simulink library "controls_module_lib"  (R2024b)
settings: Solver=VariableStepAuto  StartTime=0.0  StopTime=10.0  RelTol=1e-3
undefined symbols (not defined in the file): j, S_NOM, SNOM, VLL, VLL_NOM
libraries: simulink x14
(part 1 of 2)
settings Model: Creator=HussamAlatrash  LastModifiedBy=HussamAlatrash

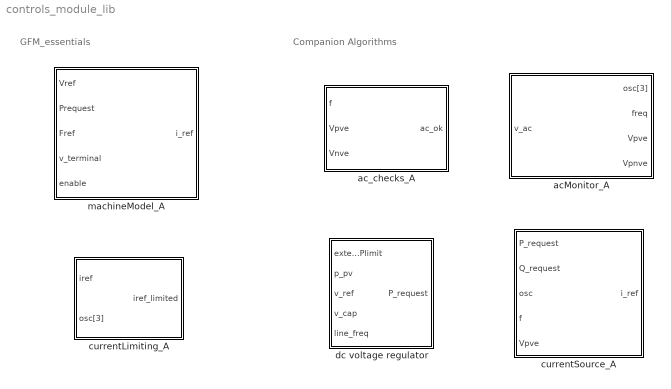
== system controls_module_lib ==
  note: Companion Algorithms
  note: GFM_essentials
  acMonitor_A : Subsystem  mask{VllRated=VLL, nominalFrequency=60}
      mask prompts: VllRated "Rated line-to-line voltage (V)"; nominalFrequency "Nominal line frequency (Hz)"
  ac_checks_A : Subsystem  mask{VllRated=1, nominalFrequency=60, tRequalify=5, T_CNTL=1e-3}
      mask prompts: VllRated "Rated line-to-line voltage (V)"; nominalFrequency "Nominal line frequency (Hz)"; tRequalify "Reconnection time (sec)"; T_CNTL "Operating sample time"
  currentLimiting_A : Subsystem  mask{IRated=SNOM/(sqrt(3)*VLL), RmsLimit=1.5, peakSoftLimit=2.6, peakHardLimit=3.5}
      mask prompts: IRated "Rated current (A)"; RmsLimit "Rms Current Limit (pu)"; peakSoftLimit "Soft peak limit (pu)"; peakHardLimit "Hard peak limit (pu)"
  currentSource_A : Subsystem  mask{VllRated=VLL_NOM, SRated=S_NOM, nominalFrequency=60, Plimit=1, Qlimit=0.5}
      mask prompts: VllRated "Rated line-to-line voltage (V)"; SRated "Rated power (VA)"; nominalFrequency "Nominal line frequency (Hz)"; Plimit "Real power request limit (pu)"; Qlimit "Reactive power request limit (pu)"
  dc voltage regulator : Subsystem  mask{kpFast=300, kpSlow=0.0, pRequestMax=1.2*S_NOM, pRequestMin=-1.2*S_NOM, pLimitExternalMinimum=0.05*SNOM}
      mask prompts: kpFast "Proportional gain - fast path (W/V)"; kpSlow "Proportional gain - filtered (slow) path (W/V)"; pRequestMax "Maximum power request (W)"; pRequestMin "Minimum power request (W)"; pLimitExternalMinimum "Minimum value for external power limit (W)"
  machineModel_A : Subsystem  mask{SRated=SNOM, VllRated=VLL, nominalFrequency=60, inertialConstant=2, kDroop=1, kDamper=2, Xs=0.2, rs=0.03}
      mask prompts: SRated "Rated power (VA)"; VllRated "Rated Voltage (Volts, line-to-line)"; nominalFrequency "Nominal frequency (Hz)"; inertialConstant "Inertial constant (seconds)"; kDroop "Droop gain (pu/Hz)"; kDamper "Damper gain (pu/Hz)"; Xs "Stator reactance (pu)"; rs "Stator resistance (pu)"

== system controls_module_lib/acMonitor_A ==
  v_ac : Inport
  Analyzer_V : Subsystem
  PLL_3ph : Subsystem
  to_pu : Gain  Gain=1/VllRated
  osc[3] : Outport
  freq : Outport  Port=2
  Vpve : Outport  Port=3
  Vpnve : Outport  Port=4
  wires:
  PLL_3ph/1(osc[3]) -> Analyzer_V/2(osc[3]), osc[3]/1
  PLL_3ph/2(freq) -> freq/1
  v_ac/1 -> Analyzer_V/1(in[3]), to_pu/1
  to_pu/1 -> PLL_3ph/1(ref)
  Analyzer_V/3(Pve) -> Vpve/1
  Analyzer_V/4(Nve) -> Vpnve/1

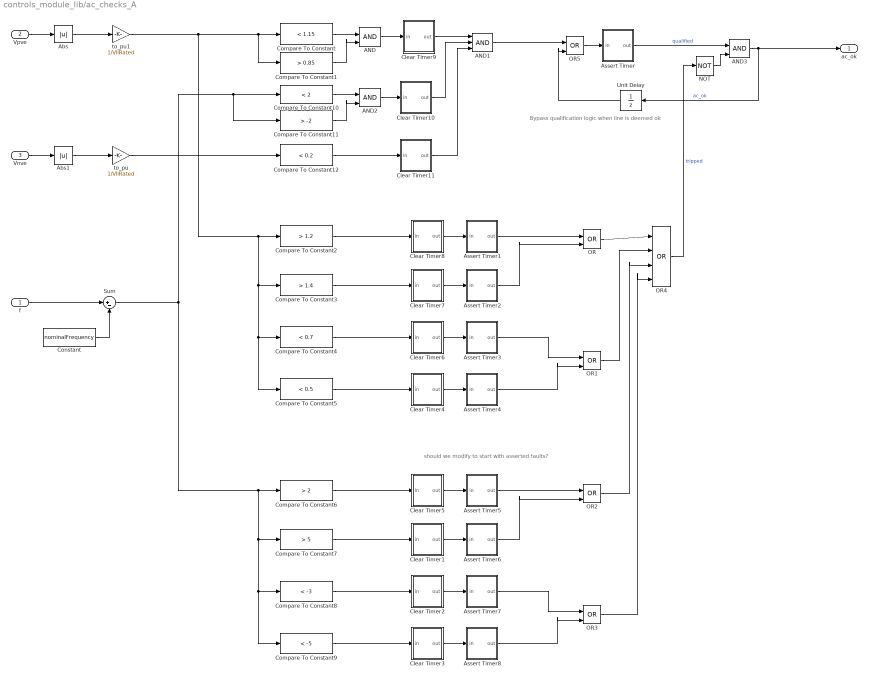
== system controls_module_lib/ac_checks_A ==
  note: should we modify to start with asserted faults?
  note: Bypass qualification logic when line is deemed ok
  f : Inport
  Vpve : Inport  Port=2
  Vnve : Inport  Port=3
  AND : Logic  IconShape=distinctive  AllPortsSameDT=off  OutDataTypeStr=boolean
  AND1 : Logic  Inputs=3  IconShape=distinctive  AllPortsSameDT=off  OutDataTypeStr=boolean
  AND2 : Logic  IconShape=distinctive  AllPortsSameDT=off  OutDataTypeStr=boolean
  AND3 : Logic  IconShape=distinctive  AllPortsSameDT=off  OutDataTypeStr=boolean
  Abs : Abs  SaturateOnIntegerOverflow=off
  Abs1 : Abs  SaturateOnIntegerOverflow=off
  Assert Timer : Subsystem  mask{T_STEP=T_CNTL, TIMEOUT=tRequalify}
      mask prompts: T_STEP "Time step"
  Assert Timer1 : Subsystem  mask{T_STEP=T_CNTL, TIMEOUT=60}
      mask prompts: T_STEP "Time step"
  Assert Timer2 : Subsystem  mask{T_STEP=T_CNTL, TIMEOUT=10}
      mask prompts: T_STEP "Time step"
  Assert Timer3 : Subsystem  mask{T_STEP=T_CNTL, TIMEOUT=60}
      mask prompts: T_STEP "Time step"
  Assert Timer4 : Subsystem  mask{T_STEP=T_CNTL, TIMEOUT=10}
      mask prompts: T_STEP "Time step"
  Assert Timer5 : Subsystem  mask{T_STEP=T_CNTL, TIMEOUT=60}
      mask prompts: T_STEP "Time step"
  Assert Timer6 : Subsystem  mask{T_STEP=T_CNTL, TIMEOUT=10}
      mask prompts: T_STEP "Time step"
  Assert Timer7 : Subsystem  mask{T_STEP=T_CNTL, TIMEOUT=60}
      mask prompts: T_STEP "Time step"
  Assert Timer8 : Subsystem  mask{T_STEP=T_CNTL, TIMEOUT=10}
      mask prompts: T_STEP "Time step"
  Clear Timer1 : Subsystem  mask{T_STEP=T_CNTL, TIMEOUT=0.1, TIMER_INIT=0.1}
      mask prompts: T_STEP "Time step"; TIMER_INIT "Timer initial value"
  Clear Timer10 : Subsystem  mask{T_STEP=T_CNTL, TIMEOUT=0.1, TIMER_INIT=0}
      mask prompts: T_STEP "Time step"; TIMER_INIT "Timer initial value"
  Clear Timer11 : Subsystem  mask{T_STEP=T_CNTL, TIMEOUT=0.1, TIMER_INIT=0}
      mask prompts: T_STEP "Time step"; TIMER_INIT "Timer initial value"
  Clear Timer2 : Subsystem  mask{T_STEP=T_CNTL, TIMEOUT=0.1, TIMER_INIT=0.1}
      mask prompts: T_STEP "Time step"; TIMER_INIT "Timer initial value"
  Clear Timer3 : Subsystem  mask{T_STEP=T_CNTL, TIMEOUT=0.1, TIMER_INIT=0.1}
      mask prompts: T_STEP "Time step"; TIMER_INIT "Timer initial value"
  Clear Timer4 : Subsystem  mask{T_STEP=T_CNTL, TIMEOUT=0.1, TIMER_INIT=0}
      mask prompts: T_STEP "Time step"; TIMER_INIT "Timer initial value"
  Clear Timer5 : Subsystem  mask{T_STEP=T_CNTL, TIMEOUT=0.1, TIMER_INIT=0.1}
      mask prompts: T_STEP "Time step"; TIMER_INIT "Timer initial value"
  Clear Timer6 : Subsystem  mask{T_STEP=T_CNTL, TIMEOUT=0.1, TIMER_INIT=0}
      mask prompts: T_STEP "Time step"; TIMER_INIT "Timer initial value"
  Clear Timer7 : Subsystem  mask{T_STEP=T_CNTL, TIMEOUT=0.1, TIMER_INIT=0}
      mask prompts: T_STEP "Time step"; TIMER_INIT "Timer initial value"
  Clear Timer8 : Subsystem  mask{T_STEP=T_CNTL, TIMEOUT=0.1, TIMER_INIT=0}
      mask prompts: T_STEP "Time step"; TIMER_INIT "Timer initial value"
  Clear Timer9 : Subsystem  mask{T_STEP=T_CNTL, TIMEOUT=0.1, TIMER_INIT=0}
      mask prompts: T_STEP "Time step"; TIMER_INIT "Timer initial value"
  Compare To Constant : simulink/Logic and Bit Operations/Compare To Constant  relop=<  const=1.15  OutDataTypeStr=boolean
  Compare To Constant1 : simulink/Logic and Bit Operations/Compare To Constant  relop=>  const=0.85  OutDataTypeStr=boolean
  Compare To Constant10 : simulink/Logic and Bit Operations/Compare To Constant  relop=<  const=2  OutDataTypeStr=boolean
  Compare To Constant11 : simulink/Logic and Bit Operations/Compare To Constant  relop=>  const=-2  OutDataTypeStr=boolean
  Compare To Constant12 : simulink/Logic and Bit Operations/Compare To Constant  relop=<  const=0.2  OutDataTypeStr=boolean
  Compare To Constant2 : simulink/Logic and Bit Operations/Compare To Constant  relop=>  const=1.2  OutDataTypeStr=boolean
  Compare To Constant3 : simulink/Logic and Bit Operations/Compare To Constant  relop=>  const=1.4  OutDataTypeStr=boolean
  Compare To Constant4 : simulink/Logic and Bit Operations/Compare To Constant  relop=<  const=0.7  OutDataTypeStr=boolean
  Compare To Constant5 : simulink/Logic and Bit Operations/Compare To Constant  relop=<  const=0.5  OutDataTypeStr=boolean
  Compare To Constant6 : simulink/Logic and Bit Operations/Compare To Constant  relop=>  const=2  OutDataTypeStr=boolean
  Compare To Constant7 : simulink/Logic and Bit Operations/Compare To Constant  relop=>  const=5  OutDataTypeStr=boolean
  Compare To Constant8 : simulink/Logic and Bit Operations/Compare To Constant  relop=<  const=-3  OutDataTypeStr=boolean
  Compare To Constant9 : simulink/Logic and Bit Operations/Compare To Constant  relop=<  const=-5  OutDataTypeStr=boolean
  Constant : Constant  Value=nominalFrequency
  NOT : Logic  Operator=NOT  IconShape=distinctive  AllPortsSameDT=off  OutDataTypeStr=boolean
  OR{,1..3,5} (5 alike) : Logic  Operator=OR  IconShape=distinctive  AllPortsSameDT=off  OutDataTypeStr=boolean
  OR4 : Logic  Operator=OR  Inputs=4  IconShape=distinctive  AllPortsSameDT=off  OutDataTypeStr=boolean
  Sum : Sum  Inputs=|+-
  Unit Delay : UnitDelay  SampleTime=T_CNTL  HasFrameUpgradeWarning=on
  to_pu : Gain  Gain=1/VllRated
  to_pu1 : Gain  Gain=1/VllRated
  ac_ok : Outport
  wires:
  OR2/1 -> OR4/3
  AND3/1 -> ac_ok/1, Unit Delay/1  "ac_ok"
  Clear Timer4/1(out) -> Assert Timer4/1(in)
  OR/1 -> OR4/1
  Clear Timer9/1(out) -> AND1/1
  Compare To Constant10/1 -> AND2/1
  Assert Timer2/1(out) -> OR/2
  OR4/1 -> NOT/1  "tripped"
  Sum/1 -> Compare To Constant6/1, Compare To Constant7/1, Compare To Constant8/1, Compare To Constant9/1, Compare To Constant10/1, Compare To Constant11/1
  Clear Timer7/1(out) -> Assert Timer2/1(in)
  Vpve/1 -> Abs/1
  Clear Timer3/1(out) -> Assert Timer8/1(in)
  Clear Timer10/1(out) -> AND1/2
  Compare To Constant7/1 -> Clear Timer1/1(in)
  Compare To Constant5/1 -> Clear Timer4/1(in)
  AND/1 -> Clear Timer9/1(in)
  Clear Timer2/1(out) -> Assert Timer7/1(in)
  OR1/1 -> OR4/2
  Compare To Constant8/1 -> Clear Timer2/1(in)
  AND1/1 -> OR5/1
  Clear Timer6/1(out) -> Assert Timer3/1(in)
  Assert Timer6/1(out) -> OR2/2
  Compare To Constant4/1 -> Clear Timer6/1(in)
  Compare To Constant11/1 -> AND2/2
  Compare To Constant9/1 -> Clear Timer3/1(in)
  AND2/1 -> Clear Timer10/1(in)
  Compare To Constant3/1 -> Clear Timer7/1(in)
  Compare To Constant/1 -> AND/1
  Assert Timer3/1(out) -> OR1/1
  NOT/1 -> AND3/2
  Vnve/1 -> Abs1/1
  Assert Timer8/1(out) -> OR3/2
  Assert Timer7/1(out) -> OR3/1
  Clear Timer8/1(out) -> Assert Timer1/1(in)
  Clear Timer1/1(out) -> Assert Timer6/1(in)
  Compare To Constant6/1 -> Clear Timer5/1(in)
  Clear Timer5/1(out) -> Assert Timer5/1(in)
  Assert Timer5/1(out) -> OR2/1
  Assert Timer4/1(out) -> OR1/2
  OR3/1 -> OR4/4
  Assert Timer/1(out) -> AND3/1  "qualified"
  Compare To Constant1/1 -> AND/2
  Compare To Constant2/1 -> Clear Timer8/1(in)
  OR5/1 -> Assert Timer/1(in)
  Clear Timer11/1(out) -> AND1/3
  Compare To Constant12/1 -> Clear Timer11/1(in)
  Assert Timer1/1(out) -> OR/1
  Unit Delay/1 -> OR5/2
  Abs/1 -> to_pu1/1
  Abs1/1 -> to_pu/1
  to_pu1/1 -> Compare To Constant1/1, Compare To Constant/1, Compare To Constant5/1, Compare To Constant4/1, Compare To Constant3/1, Compare To Constant2/1
  to_pu/1 -> Compare To Constant12/1
  f/1 -> Sum/1
  Constant/1 -> Sum/2

== system controls_module_lib/currentLimiting_A ==
  iref : Inport
  osc[3] : Inport  Port=2
  Analyzer_I : Subsystem
  Sum2 : Sum  Inputs=|+-
  excess_sink : Subsystem
  soft_saturation : Subsystem  mask{soft_limit=peakSoftLimit*IRated, hard_limit=peakHardLimit*IRated}
      mask prompts: soft_limit "Soft limit"; hard_limit "Hard limit"
  iref_limited : Outport
  wires:
  Sum2/1 -> soft_saturation/1(in)
  osc[3]/1 -> excess_sink/2(osc[3]), Analyzer_I/2(osc[3])
  iref/1 -> Sum2/1, Analyzer_I/1(in[3])
  excess_sink/1(i_excess[3]) -> Sum2/2
  Analyzer_I/1(fund[3]) -> excess_sink/1(I_total[3])  "I_total[3]"
  soft_saturation/1(out) -> iref_limited/1

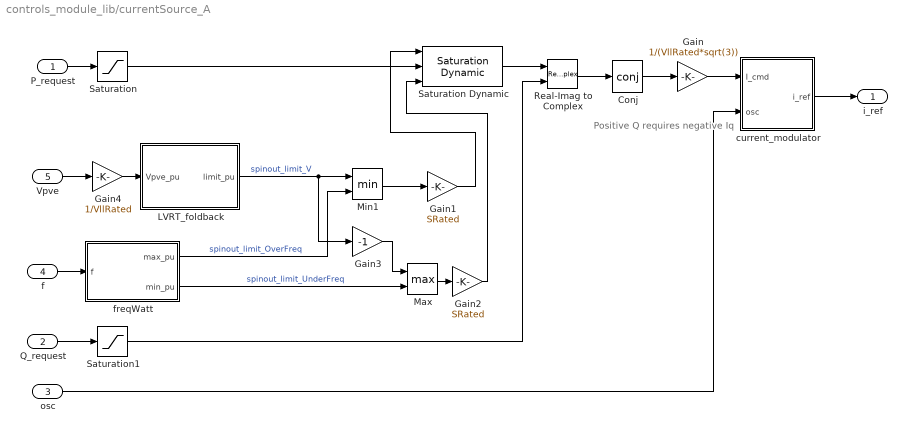
== system controls_module_lib/currentSource_A ==
  note: Positive Q requires negative Iq
  P_request : Inport
  Q_request : Inport  Port=2
  osc : Inport  Port=3
  f : Inport  Port=4
  Vpve : Inport  Port=5
  Conj : Math  Operator=conj
  Gain : Gain  Gain=1/(VllRated*sqrt(3))
  Gain1 : Gain  Gain=SRated
  Gain2 : Gain  Gain=SRated
  Gain3 : Gain  Gain=-1
  Gain4 : Gain  Gain=1/VllRated
  LVRT_foldback : Subsystem
  Max : MinMax  Function=max  Inputs=2
  Min1 : MinMax  Inputs=2
  Real-Imag to Complex : RealImagToComplex
  Saturation : Saturate  UpperLimit=Plimit*SRated  LowerLimit=-Plimit*SRated
  Saturation Dynamic : simulink/Discontinuities/Saturation Dynamic  OutMin=[]  OutMax=[]  OutDataTypeStr=Inherit: Same as second input  OutDataType=fixdt(1, 16)  OutScaling=2^-10  DoSatur=off
  Saturation1 : Saturate  UpperLimit=Qlimit*SRated  LowerLimit=-Qlimit*SRated
  current_modulator : Subsystem
  freqWatt : Subsystem
  i_ref : Outport
  wires:
  LVRT_foldback/1(limit_pu) -> Min1/1, Gain3/1  "spinout_limit_V"
  Vpve/1 -> Gain4/1
  Min1/1 -> Gain1/1
  f/1 -> freqWatt/1(f)
  freqWatt/1(max_pu) -> Min1/2  "spinout_limit_OverFreq"
  current_modulator/1(i_ref) -> i_ref/1
  Q_request/1 -> Saturation1/1
  P_request/1 -> Saturation/1
  osc/1 -> current_modulator/2(osc)
  Gain4/1 -> LVRT_foldback/1(Vpve_pu)
  Saturation Dynamic/1 -> Real-Imag to Complex/1
  Gain1/1 -> Saturation Dynamic/1
  Real-Imag to Complex/1 -> Conj/1
  Conj/1 -> Gain/1
  Gain/1 -> current_modulator/1(I_cmd)
  Saturation/1 -> Saturation Dynamic/2
  Saturation1/1 -> Real-Imag to Complex/2
  Max/1 -> Gain2/1
  freqWatt/2(min_pu) -> Max/2  "spinout_limit_UnderFreq"
  Gain2/1 -> Saturation Dynamic/3
  Gain3/1 -> Max/1

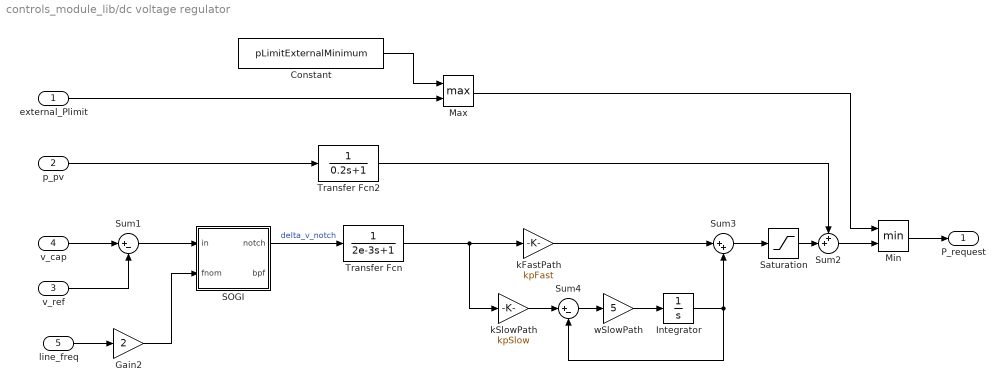
== system controls_module_lib/dc voltage regulator ==
  external_Plimit : Inport
  p_pv : Inport  Port=2
  v_ref : Inport  Port=3
  v_cap : Inport  Port=4
  line_freq : Inport  Port=5
  Constant : Constant  Value=pLimitExternalMinimum
  Gain2 : Gain  Gain=2
  Integrator : Integrator  LimitOutput=on  UpperSaturationLimit=0.4  LowerSaturationLimit=-0.1
  Max : MinMax  Function=max  Inputs=2
  Min : MinMax  Inputs=2
  SOGI : Subsystem
  Saturation : Saturate  UpperLimit=pRequestMax  LowerLimit=pRequestMin
  Sum1 : Sum  Inputs=|+-
  Sum2 : Sum  Inputs=++|
  Sum3 : Sum  Inputs=|++
  Sum4 : Sum  Inputs=|+-
  Transfer Fcn : TransferFcn  Denominator=[2e-3 1]
  Transfer Fcn2 : TransferFcn  Denominator=[0.2 1]
  kFastPath : Gain  Gain=kpFast
  kSlowPath : Gain  Gain=kpSlow
  wSlowPath : Gain  Gain=5
  P_request : Outport
  wires:
  Constant/1 -> Max/1
  external_Plimit/1 -> Max/2
  Max/1 -> Min/1
  Min/1 -> P_request/1
  v_ref/1 -> Sum1/2
  Sum2/1 -> Min/2
  Gain2/1 -> SOGI/2(fnom)
  SOGI/1(notch) -> Transfer Fcn/1  "delta_v_notch"
  v_cap/1 -> Sum1/1
  p_pv/1 -> Transfer Fcn2/1
  Transfer Fcn/1 -> kSlowPath/1, kFastPath/1
  kFastPath/1 -> Sum3/1
  Sum3/1 -> Saturation/1
  kSlowPath/1 -> Sum4/1
  Transfer Fcn2/1 -> Sum2/1
  line_freq/1 -> Gain2/1
  Integrator/1 -> Sum4/2, Sum3/2
  Saturation/1 -> Sum2/2
  wSlowPath/1 -> Integrator/1
  Sum4/1 -> wSlowPath/1
  Sum1/1 -> SOGI/1(in)

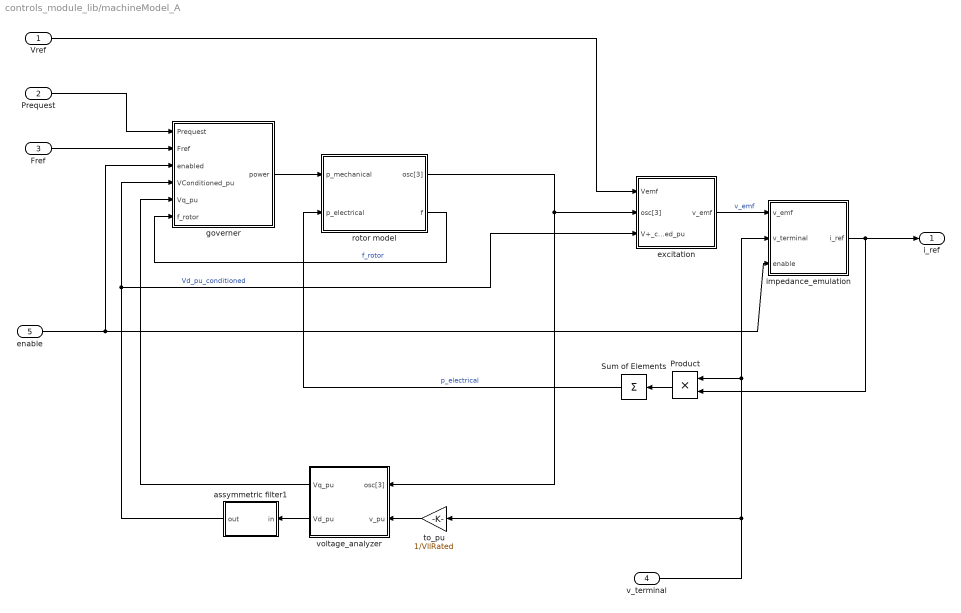
== system controls_module_lib/machineModel_A ==
  Vref : Inport
  Prequest : Inport  Port=2
  Fref : Inport  Port=3
  v_terminal : Inport  Port=4
  enable : Inport  Port=5
  Product : Product
  Sum of Elements : Sum  Inputs=+
  assymmetric filter1 : Subsystem
  excitation : Subsystem
  governer : Subsystem
  impedance_emulation : Subsystem
  rotor model : Subsystem
  to_pu : Gain  Gain=1/VllRated
  voltage_analyzer : Subsystem
  i_ref : Outport
  wires:
  excitation/1(v_emf) -> impedance_emulation/1(v_emf)  "v_emf"
  rotor model/1(osc[3]) -> excitation/2(osc[3]), voltage_analyzer/1(osc[3])
  Product/1 -> Sum of Elements/1
  Sum of Elements/1 -> rotor model/2(p_electrical)  "p_electrical"
  governer/1(power) -> rotor model/1(p_mechanical)
  voltage_analyzer/2(Vd_pu) -> assymmetric filter1/1(in)
  Prequest/1 -> governer/1(Prequest)
  impedance_emulation/1(i_ref) -> i_ref/1, Product/2
  to_pu/1 -> voltage_analyzer/2(v_pu)
  v_terminal/1 -> to_pu/1, impedance_emulation/2(v_terminal), Product/1
  voltage_analyzer/1(Vq_pu) -> governer/5(Vq_pu)
  rotor model/2(f) -> governer/6(f_rotor)  "f_rotor"
  assymmetric filter1/1(out) -> excitation/3(V+_conditioned_pu), governer/4(VConditioned_pu)  "Vd_pu_conditioned"
  enable/1 -> governer/3(enabled), impedance_emulation/3(enable)
  Fref/1 -> governer/2(Fref)
  Vref/1 -> excitation/1(Vemf)

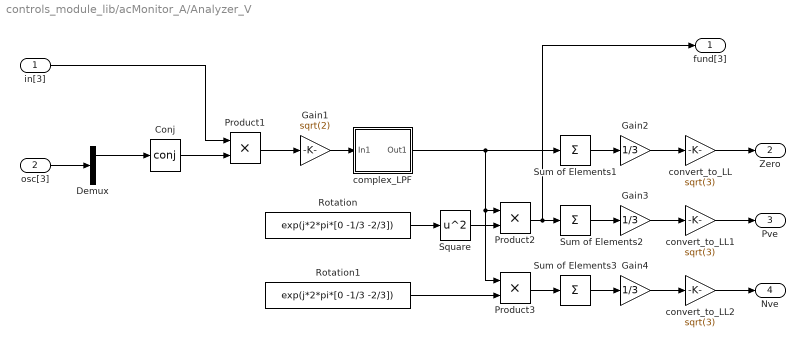
== system controls_module_lib/acMonitor_A/Analyzer_V ==
  in[3] : Inport
  osc[3] : Inport  Port=2
  Conj : Math  Operator=conj
  Demux : Demux  Outputs=3
  Gain1 : Gain  Gain=sqrt(2)
  Gain2 : Gain  Gain=1/3
  Gain3 : Gain  Gain=1/3
  Gain4 : Gain  Gain=1/3
  Product1 : Product
  Product2 : Product
  Product3 : Product
  Rotation : Constant  Value=exp(j*2*pi*[0 -1/3 -2/3])
  Rotation1 : Constant  Value=exp(j*2*pi*[0 -1/3 -2/3])
  Square : Math  Operator=square
  Sum of Elements1 : Sum  Inputs=+
  Sum of Elements2 : Sum  Inputs=+
  Sum of Elements3 : Sum  Inputs=+
  complex_LPF : Subsystem  mask{tau=0.05}
      mask prompts: tau "Time constant"
  convert_to_LL : Gain  Gain=sqrt(3)
  convert_to_LL1 : Gain  Gain=sqrt(3)
  convert_to_LL2 : Gain  Gain=sqrt(3)
  fund[3] : Outport
  Zero : Outport  Port=2
  Pve : Outport  Port=3
  Nve : Outport  Port=4
  wires:
  Gain4/1 -> convert_to_LL2/1
  Product2/1 -> fund[3]/1, Sum of Elements2/1
  complex_LPF/1(Out1) -> Product3/1, Product2/1, Sum of Elements1/1
  Product1/1 -> Gain1/1
  Product3/1 -> Sum of Elements3/1
  Gain1/1 -> complex_LPF/1(In1)
  Demux/1 -> Conj/1
  Rotation/1 -> Square/1
  Rotation1/1 -> Product3/2
  Sum of Elements2/1 -> Gain3/1
  Conj/1 -> Product1/2
  Sum of Elements1/1 -> Gain2/1
  Square/1 -> Product2/2
  Sum of Elements3/1 -> Gain4/1
  osc[3]/1 -> Demux/1
  Gain3/1 -> convert_to_LL1/1
  Gain2/1 -> convert_to_LL/1
  in[3]/1 -> Product1/1
  convert_to_LL/1 -> Zero/1
  convert_to_LL1/1 -> Pve/1
  convert_to_LL2/1 -> Nve/1

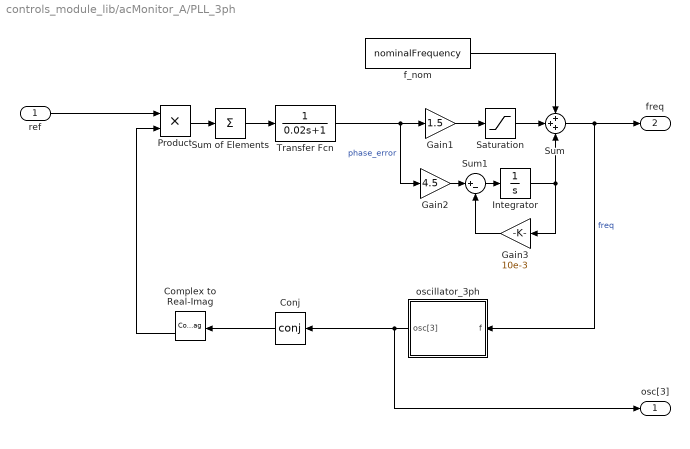
== system controls_module_lib/acMonitor_A/PLL_3ph ==
  ref : Inport
  Complex to Real-Imag : ComplexToRealImag
  Conj : Math  Operator=conj
  Gain1 : Gain  Gain=1.5
  Gain2 : Gain  Gain=4.5
  Gain3 : Gain  Gain=10e-3
  Integrator : Integrator  LimitOutput=on  UpperSaturationLimit=5  LowerSaturationLimit=-5
  Product : Product
  Saturation : Saturate  UpperLimit=5  LowerLimit=-5
  Sum : Sum  Inputs=+++
  Sum of Elements : Sum  Inputs=+
  Sum1 : Sum  Inputs=|+-
  Transfer Fcn : TransferFcn  Denominator=[0.02 1]
  f_nom : Constant  Value=nominalFrequency
  oscillator_3ph : Subsystem
  osc[3] : Outport
  freq : Outport  Port=2
  wires:
  f_nom/1 -> Sum/1
  Gain3/1 -> Sum1/2
  Sum of Elements/1 -> Transfer Fcn/1
  Transfer Fcn/1 -> Gain2/1, Gain1/1  "phase_error"
  Saturation/1 -> Sum/2
  Product/1 -> Sum of Elements/1
  Sum/1 -> freq/1, oscillator_3ph/1(f)  "freq"
  oscillator_3ph/1(osc[3]) -> Conj/1, osc[3]/1
  Gain2/1 -> Sum1/1
  Complex to Real-Imag/2 -> Product/2
  Sum1/1 -> Integrator/1
  Integrator/1 -> Gain3/1, Sum/3
  ref/1 -> Product/1
  Conj/1 -> Complex to Real-Imag/1
  Gain1/1 -> Saturation/1

== system controls_module_lib/ac_checks_A/Assert Timer ==
  in : Inport
  Constant : Constant  Value=T_STEP
  Constant1 : Constant  Value=0
  Constant2 : Constant  Value=TIMEOUT
  Min2 : MinMax  Inputs=2
  Relational Operator : RelationalOperator  Operator=>  OutDataTypeStr=boolean  RndMeth=Simplest  InputSameDT=off
  Sum2 : Sum  Inputs=|++
  Switch : Switch  Criteria=u2 > Threshold  SaturateOnIntegerOverflow=off  InputSameDT=off
  Unit Delay : UnitDelay  SampleTime=T_STEP  HasFrameUpgradeWarning=on
  out : Outport
  wires:
  Sum2/1 -> Relational Operator/1, Min2/1
  Constant2/1 -> Min2/2, Relational Operator/2
  Constant/1 -> Sum2/1
  Min2/1 -> Switch/1
  Constant1/1 -> Switch/3
  Unit Delay/1 -> Sum2/2
  in/1 -> Switch/2
  Switch/1 -> Unit Delay/1
  Relational Operator/1 -> out/1

== system controls_module_lib/ac_checks_A/Assert Timer1 ==
  in : Inport
  Constant : Constant  Value=T_STEP
  Constant1 : Constant  Value=0
  Constant2 : Constant  Value=TIMEOUT
  Min2 : MinMax  Inputs=2
  Relational Operator : RelationalOperator  Operator=>  OutDataTypeStr=boolean  RndMeth=Simplest  InputSameDT=off
  Sum2 : Sum  Inputs=|++
  Switch : Switch  Criteria=u2 > Threshold  SaturateOnIntegerOverflow=off  InputSameDT=off
  Unit Delay : UnitDelay  SampleTime=T_STEP  HasFrameUpgradeWarning=on
  out : Outport
  wires:
  Relational Operator/1 -> out/1
  Switch/1 -> Unit Delay/1
  in/1 -> Switch/2
  Unit Delay/1 -> Sum2/2
  Constant1/1 -> Switch/3
  Min2/1 -> Switch/1
  Constant/1 -> Sum2/1
  Constant2/1 -> Relational Operator/2, Min2/2
  Sum2/1 -> Min2/1, Relational Operator/1

== system controls_module_lib/ac_checks_A/Assert Timer2 ==
  in : Inport
  Constant : Constant  Value=T_STEP
  Constant1 : Constant  Value=0
  Constant2 : Constant  Value=TIMEOUT
  Min2 : MinMax  Inputs=2
  Relational Operator : RelationalOperator  Operator=>  OutDataTypeStr=boolean  RndMeth=Simplest  InputSameDT=off
  Sum2 : Sum  Inputs=|++
  Switch : Switch  Criteria=u2 > Threshold  SaturateOnIntegerOverflow=off  InputSameDT=off
  Unit Delay : UnitDelay  SampleTime=T_STEP  HasFrameUpgradeWarning=on
  out : Outport
  wires:
  Sum2/1 -> Relational Operator/1, Min2/1
  Constant2/1 -> Min2/2, Relational Operator/2
  Constant/1 -> Sum2/1
  Min2/1 -> Switch/1
  Constant1/1 -> Switch/3
  Unit Delay/1 -> Sum2/2
  in/1 -> Switch/2
  Switch/1 -> Unit Delay/1
  Relational Operator/1 -> out/1

== system controls_module_lib/ac_checks_A/Assert Timer3 ==
  in : Inport
  Constant : Constant  Value=T_STEP
  Constant1 : Constant  Value=0
  Constant2 : Constant  Value=TIMEOUT
  Min2 : MinMax  Inputs=2
  Relational Operator : RelationalOperator  Operator=>  OutDataTypeStr=boolean  RndMeth=Simplest  InputSameDT=off
  Sum2 : Sum  Inputs=|++
  Switch : Switch  Criteria=u2 > Threshold  SaturateOnIntegerOverflow=off  InputSameDT=off
  Unit Delay : UnitDelay  SampleTime=T_STEP  HasFrameUpgradeWarning=on
  out : Outport
  wires:
  Relational Operator/1 -> out/1
  Switch/1 -> Unit Delay/1
  in/1 -> Switch/2
  Unit Delay/1 -> Sum2/2
  Constant1/1 -> Switch/3
  Min2/1 -> Switch/1
  Constant/1 -> Sum2/1
  Constant2/1 -> Relational Operator/2, Min2/2
  Sum2/1 -> Min2/1, Relational Operator/1

== system controls_module_lib/ac_checks_A/Assert Timer4 ==
  in : Inport
  Constant : Constant  Value=T_STEP
  Constant1 : Constant  Value=0
  Constant2 : Constant  Value=TIMEOUT
  Min2 : MinMax  Inputs=2
  Relational Operator : RelationalOperator  Operator=>  OutDataTypeStr=boolean  RndMeth=Simplest  InputSameDT=off
  Sum2 : Sum  Inputs=|++
  Switch : Switch  Criteria=u2 > Threshold  SaturateOnIntegerOverflow=off  InputSameDT=off
  Unit Delay : UnitDelay  SampleTime=T_STEP  HasFrameUpgradeWarning=on
  out : Outport
  wires:
  Sum2/1 -> Relational Operator/1, Min2/1
  Constant2/1 -> Min2/2, Relational Operator/2
  Constant/1 -> Sum2/1
  Min2/1 -> Switch/1
  Constant1/1 -> Switch/3
  Unit Delay/1 -> Sum2/2
  in/1 -> Switch/2
  Switch/1 -> Unit Delay/1
  Relational Operator/1 -> out/1

== system controls_module_lib/ac_checks_A/Assert Timer5 ==
  in : Inport
  Constant : Constant  Value=T_STEP
  Constant1 : Constant  Value=0
  Constant2 : Constant  Value=TIMEOUT
  Min2 : MinMax  Inputs=2
  Relational Operator : RelationalOperator  Operator=>  OutDataTypeStr=boolean  RndMeth=Simplest  InputSameDT=off
  Sum2 : Sum  Inputs=|++
  Switch : Switch  Criteria=u2 > Threshold  SaturateOnIntegerOverflow=off  InputSameDT=off
  Unit Delay : UnitDelay  SampleTime=T_STEP  HasFrameUpgradeWarning=on
  out : Outport
  wires:
  Sum2/1 -> Relational Operator/1, Min2/1
  Constant2/1 -> Min2/2, Relational Operator/2
  Constant/1 -> Sum2/1
  Min2/1 -> Switch/1
  Constant1/1 -> Switch/3
  Unit Delay/1 -> Sum2/2
  in/1 -> Switch/2
  Switch/1 -> Unit Delay/1
  Relational Operator/1 -> out/1

== system controls_module_lib/ac_checks_A/Assert Timer6 ==
  in : Inport
  Constant : Constant  Value=T_STEP
  Constant1 : Constant  Value=0
  Constant2 : Constant  Value=TIMEOUT
  Min2 : MinMax  Inputs=2
  Relational Operator : RelationalOperator  Operator=>  OutDataTypeStr=boolean  RndMeth=Simplest  InputSameDT=off
  Sum2 : Sum  Inputs=|++
  Switch : Switch  Criteria=u2 > Threshold  SaturateOnIntegerOverflow=off  InputSameDT=off
  Unit Delay : UnitDelay  SampleTime=T_STEP  HasFrameUpgradeWarning=on
  out : Outport
  wires:
  Relational Operator/1 -> out/1
  Switch/1 -> Unit Delay/1
  in/1 -> Switch/2
  Unit Delay/1 -> Sum2/2
  Constant1/1 -> Switch/3
  Min2/1 -> Switch/1
  Constant/1 -> Sum2/1
  Constant2/1 -> Relational Operator/2, Min2/2
  Sum2/1 -> Min2/1, Relational Operator/1

== system controls_module_lib/ac_checks_A/Assert Timer7 ==
  in : Inport
  Constant : Constant  Value=T_STEP
  Constant1 : Constant  Value=0
  Constant2 : Constant  Value=TIMEOUT
  Min2 : MinMax  Inputs=2
  Relational Operator : RelationalOperator  Operator=>  OutDataTypeStr=boolean  RndMeth=Simplest  InputSameDT=off
  Sum2 : Sum  Inputs=|++
  Switch : Switch  Criteria=u2 > Threshold  SaturateOnIntegerOverflow=off  InputSameDT=off
  Unit Delay : UnitDelay  SampleTime=T_STEP  HasFrameUpgradeWarning=on
  out : Outport
  wires:
  Sum2/1 -> Relational Operator/1, Min2/1
  Constant2/1 -> Min2/2, Relational Operator/2
  Constant/1 -> Sum2/1
  Min2/1 -> Switch/1
  Constant1/1 -> Switch/3
  Unit Delay/1 -> Sum2/2
  in/1 -> Switch/2
  Switch/1 -> Unit Delay/1
  Relational Operator/1 -> out/1

== system controls_module_lib/ac_checks_A/Assert Timer8 ==
  in : Inport
  Constant : Constant  Value=T_STEP
  Constant1 : Constant  Value=0
  Constant2 : Constant  Value=TIMEOUT
  Min2 : MinMax  Inputs=2
  Relational Operator : RelationalOperator  Operator=>  OutDataTypeStr=boolean  RndMeth=Simplest  InputSameDT=off
  Sum2 : Sum  Inputs=|++
  Switch : Switch  Criteria=u2 > Threshold  SaturateOnIntegerOverflow=off  InputSameDT=off
  Unit Delay : UnitDelay  SampleTime=T_STEP  HasFrameUpgradeWarning=on
  out : Outport
  wires:
  Relational Operator/1 -> out/1
  Switch/1 -> Unit Delay/1
  in/1 -> Switch/2
  Unit Delay/1 -> Sum2/2
  Constant1/1 -> Switch/3
  Min2/1 -> Switch/1
  Constant/1 -> Sum2/1
  Constant2/1 -> Relational Operator/2, Min2/2
  Sum2/1 -> Min2/1, Relational Operator/1

== system controls_module_lib/ac_checks_A/Clear Timer1 ==
  in : Inport
  Constant : Constant  Value=T_STEP
  Constant1 : Constant  Value=0
  Constant2 : Constant  Value=TIMEOUT
  Min2 : MinMax  Function=max  Inputs=2
  Relational Operator : RelationalOperator  Operator=>  OutDataTypeStr=boolean  RndMeth=Simplest  InputSameDT=off
  Sum2 : Sum  Inputs=|-+
  Switch : Switch  Criteria=u2 > Threshold  SaturateOnIntegerOverflow=off  InputSameDT=off
  Unit Delay : UnitDelay  InitialCondition=TIMER_INIT  SampleTime=T_STEP  HasFrameUpgradeWarning=on
  out : Outport
  wires:
  Constant2/1 -> Switch/1
  Sum2/1 -> Relational Operator/1, Min2/1
  Constant/1 -> Sum2/1
  Min2/1 -> Switch/3
  Constant1/1 -> Min2/2, Relational Operator/2
  Unit Delay/1 -> Sum2/2
  in/1 -> Switch/2
  Switch/1 -> Unit Delay/1
  Relational Operator/1 -> out/1

== system controls_module_lib/ac_checks_A/Clear Timer10 ==
  in : Inport
  Constant : Constant  Value=T_STEP
  Constant1 : Constant  Value=0
  Constant2 : Constant  Value=TIMEOUT
  Min2 : MinMax  Function=max  Inputs=2
  Relational Operator : RelationalOperator  Operator=>  OutDataTypeStr=boolean  RndMeth=Simplest  InputSameDT=off
  Sum2 : Sum  Inputs=|-+
  Switch : Switch  Criteria=u2 > Threshold  SaturateOnIntegerOverflow=off  InputSameDT=off
  Unit Delay : UnitDelay  InitialCondition=TIMER_INIT  SampleTime=T_STEP  HasFrameUpgradeWarning=on
  out : Outport
  wires:
  Constant2/1 -> Switch/1
  Sum2/1 -> Relational Operator/1, Min2/1
  Constant/1 -> Sum2/1
  Min2/1 -> Switch/3
  Constant1/1 -> Min2/2, Relational Operator/2
  Unit Delay/1 -> Sum2/2
  in/1 -> Switch/2
  Switch/1 -> Unit Delay/1
  Relational Operator/1 -> out/1

== system controls_module_lib/ac_checks_A/Clear Timer11 ==
  in : Inport
  Constant : Constant  Value=T_STEP
  Constant1 : Constant  Value=0
  Constant2 : Constant  Value=TIMEOUT
  Min2 : MinMax  Function=max  Inputs=2
  Relational Operator : RelationalOperator  Operator=>  OutDataTypeStr=boolean  RndMeth=Simplest  InputSameDT=off
  Sum2 : Sum  Inputs=|-+
  Switch : Switch  Criteria=u2 > Threshold  SaturateOnIntegerOverflow=off  InputSameDT=off
  Unit Delay : UnitDelay  InitialCondition=TIMER_INIT  SampleTime=T_STEP  HasFrameUpgradeWarning=on
  out : Outport
  wires:
  Relational Operator/1 -> out/1
  Switch/1 -> Unit Delay/1
  in/1 -> Switch/2
  Unit Delay/1 -> Sum2/2
  Constant1/1 -> Relational Operator/2, Min2/2
  Min2/1 -> Switch/3
  Constant/1 -> Sum2/1
  Sum2/1 -> Min2/1, Relational Operator/1
  Constant2/1 -> Switch/1

== system controls_module_lib/ac_checks_A/Clear Timer2 ==
  in : Inport
  Constant : Constant  Value=T_STEP
  Constant1 : Constant  Value=0
  Constant2 : Constant  Value=TIMEOUT
  Min2 : MinMax  Function=max  Inputs=2
  Relational Operator : RelationalOperator  Operator=>  OutDataTypeStr=boolean  RndMeth=Simplest  InputSameDT=off
  Sum2 : Sum  Inputs=|-+
  Switch : Switch  Criteria=u2 > Threshold  SaturateOnIntegerOverflow=off  InputSameDT=off
  Unit Delay : UnitDelay  InitialCondition=TIMER_INIT  SampleTime=T_STEP  HasFrameUpgradeWarning=on
  out : Outport
  wires:
  Relational Operator/1 -> out/1
  Switch/1 -> Unit Delay/1
  in/1 -> Switch/2
  Unit Delay/1 -> Sum2/2
  Constant1/1 -> Relational Operator/2, Min2/2
  Min2/1 -> Switch/3
  Constant/1 -> Sum2/1
  Sum2/1 -> Min2/1, Relational Operator/1
  Constant2/1 -> Switch/1

== system controls_module_lib/ac_checks_A/Clear Timer3 ==
  in : Inport
  Constant : Constant  Value=T_STEP
  Constant1 : Constant  Value=0
  Constant2 : Constant  Value=TIMEOUT
  Min2 : MinMax  Function=max  Inputs=2
  Relational Operator : RelationalOperator  Operator=>  OutDataTypeStr=boolean  RndMeth=Simplest  InputSameDT=off
  Sum2 : Sum  Inputs=|-+
  Switch : Switch  Criteria=u2 > Threshold  SaturateOnIntegerOverflow=off  InputSameDT=off
  Unit Delay : UnitDelay  InitialCondition=TIMER_INIT  SampleTime=T_STEP  HasFrameUpgradeWarning=on
  out : Outport
  wires:
  Constant2/1 -> Switch/1
  Sum2/1 -> Relational Operator/1, Min2/1
  Constant/1 -> Sum2/1
  Min2/1 -> Switch/3
  Constant1/1 -> Min2/2, Relational Operator/2
  Unit Delay/1 -> Sum2/2
  in/1 -> Switch/2
  Switch/1 -> Unit Delay/1
  Relational Operator/1 -> out/1

== system controls_module_lib/ac_checks_A/Clear Timer4 ==
  in : Inport
  Constant : Constant  Value=T_STEP
  Constant1 : Constant  Value=0
  Constant2 : Constant  Value=TIMEOUT
  Min2 : MinMax  Function=max  Inputs=2
  Relational Operator : RelationalOperator  Operator=>  OutDataTypeStr=boolean  RndMeth=Simplest  InputSameDT=off
  Sum2 : Sum  Inputs=|-+
  Switch : Switch  Criteria=u2 > Threshold  SaturateOnIntegerOverflow=off  InputSameDT=off
  Unit Delay : UnitDelay  InitialCondition=TIMER_INIT  SampleTime=T_STEP  HasFrameUpgradeWarning=on
  out : Outport
  wires:
  Relational Operator/1 -> out/1
  Switch/1 -> Unit Delay/1
  in/1 -> Switch/2
  Unit Delay/1 -> Sum2/2
  Constant1/1 -> Relational Operator/2, Min2/2
  Min2/1 -> Switch/3
  Constant/1 -> Sum2/1
  Sum2/1 -> Min2/1, Relational Operator/1
  Constant2/1 -> Switch/1

== system controls_module_lib/ac_checks_A/Clear Timer5 ==
  in : Inport
  Constant : Constant  Value=T_STEP
  Constant1 : Constant  Value=0
  Constant2 : Constant  Value=TIMEOUT
  Min2 : MinMax  Function=max  Inputs=2
  Relational Operator : RelationalOperator  Operator=>  OutDataTypeStr=boolean  RndMeth=Simplest  InputSameDT=off
  Sum2 : Sum  Inputs=|-+
  Switch : Switch  Criteria=u2 > Threshold  SaturateOnIntegerOverflow=off  InputSameDT=off
  Unit Delay : UnitDelay  InitialCondition=TIMER_INIT  SampleTime=T_STEP  HasFrameUpgradeWarning=on
  out : Outport
  wires:
  Relational Operator/1 -> out/1
  Switch/1 -> Unit Delay/1
  in/1 -> Switch/2
  Unit Delay/1 -> Sum2/2
  Constant1/1 -> Relational Operator/2, Min2/2
  Min2/1 -> Switch/3
  Constant/1 -> Sum2/1
  Sum2/1 -> Min2/1, Relational Operator/1
  Constant2/1 -> Switch/1

== system controls_module_lib/ac_checks_A/Clear Timer6 ==
  in : Inport
  Constant : Constant  Value=T_STEP
  Constant1 : Constant  Value=0
  Constant2 : Constant  Value=TIMEOUT
  Min2 : MinMax  Function=max  Inputs=2
  Relational Operator : RelationalOperator  Operator=>  OutDataTypeStr=boolean  RndMeth=Simplest  InputSameDT=off
  Sum2 : Sum  Inputs=|-+
  Switch : Switch  Criteria=u2 > Threshold  SaturateOnIntegerOverflow=off  InputSameDT=off
  Unit Delay : UnitDelay  InitialCondition=TIMER_INIT  SampleTime=T_STEP  HasFrameUpgradeWarning=on
  out : Outport
  wires:
  Constant2/1 -> Switch/1
  Sum2/1 -> Relational Operator/1, Min2/1
  Constant/1 -> Sum2/1
  Min2/1 -> Switch/3
  Constant1/1 -> Min2/2, Relational Operator/2
  Unit Delay/1 -> Sum2/2
  in/1 -> Switch/2
  Switch/1 -> Unit Delay/1
  Relational Operator/1 -> out/1

== system controls_module_lib/ac_checks_A/Clear Timer7 ==
  in : Inport
  Constant : Constant  Value=T_STEP
  Constant1 : Constant  Value=0
  Constant2 : Constant  Value=TIMEOUT
  Min2 : MinMax  Function=max  Inputs=2
  Relational Operator : RelationalOperator  Operator=>  OutDataTypeStr=boolean  RndMeth=Simplest  InputSameDT=off
  Sum2 : Sum  Inputs=|-+
  Switch : Switch  Criteria=u2 > Threshold  SaturateOnIntegerOverflow=off  InputSameDT=off
  Unit Delay : UnitDelay  InitialCondition=TIMER_INIT  SampleTime=T_STEP  HasFrameUpgradeWarning=on
  out : Outport
  wires:
  Relational Operator/1 -> out/1
  Switch/1 -> Unit Delay/1
  in/1 -> Switch/2
  Unit Delay/1 -> Sum2/2
  Constant1/1 -> Relational Operator/2, Min2/2
  Min2/1 -> Switch/3
  Constant/1 -> Sum2/1
  Sum2/1 -> Min2/1, Relational Operator/1
  Constant2/1 -> Switch/1

== system controls_module_lib/ac_checks_A/Clear Timer8 ==
  in : Inport
  Constant : Constant  Value=T_STEP
  Constant1 : Constant  Value=0
  Constant2 : Constant  Value=TIMEOUT
  Min2 : MinMax  Function=max  Inputs=2
  Relational Operator : RelationalOperator  Operator=>  OutDataTypeStr=boolean  RndMeth=Simplest  InputSameDT=off
  Sum2 : Sum  Inputs=|-+
  Switch : Switch  Criteria=u2 > Threshold  SaturateOnIntegerOverflow=off  InputSameDT=off
  Unit Delay : UnitDelay  InitialCondition=TIMER_INIT  SampleTime=T_STEP  HasFrameUpgradeWarning=on
  out : Outport
  wires:
  Constant2/1 -> Switch/1
  Sum2/1 -> Relational Operator/1, Min2/1
  Constant/1 -> Sum2/1
  Min2/1 -> Switch/3
  Constant1/1 -> Min2/2, Relational Operator/2
  Unit Delay/1 -> Sum2/2
  in/1 -> Switch/2
  Switch/1 -> Unit Delay/1
  Relational Operator/1 -> out/1

== system controls_module_lib/ac_checks_A/Clear Timer9 ==
  in : Inport
  Constant : Constant  Value=T_STEP
  Constant1 : Constant  Value=0
  Constant2 : Constant  Value=TIMEOUT
  Min2 : MinMax  Function=max  Inputs=2
  Relational Operator : RelationalOperator  Operator=>  OutDataTypeStr=boolean  RndMeth=Simplest  InputSameDT=off
  Sum2 : Sum  Inputs=|-+
  Switch : Switch  Criteria=u2 > Threshold  SaturateOnIntegerOverflow=off  InputSameDT=off
  Unit Delay : UnitDelay  InitialCondition=TIMER_INIT  SampleTime=T_STEP  HasFrameUpgradeWarning=on
  out : Outport
  wires:
  Relational Operator/1 -> out/1
  Switch/1 -> Unit Delay/1
  in/1 -> Switch/2
  Unit Delay/1 -> Sum2/2
  Constant1/1 -> Relational Operator/2, Min2/2
  Min2/1 -> Switch/3
  Constant/1 -> Sum2/1
  Sum2/1 -> Min2/1, Relational Operator/1
  Constant2/1 -> Switch/1

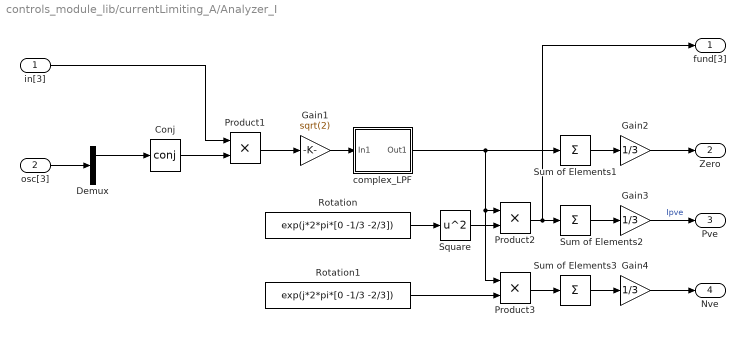
== system controls_module_lib/currentLimiting_A/Analyzer_I ==
  in[3] : Inport
  osc[3] : Inport  Port=2
  Conj : Math  Operator=conj
  Demux : Demux  Outputs=3
  Gain1 : Gain  Gain=sqrt(2)
  Gain2 : Gain  Gain=1/3
  Gain3 : Gain  Gain=1/3
  Gain4 : Gain  Gain=1/3
  Product1 : Product
  Product2 : Product
  Product3 : Product
  Rotation : Constant  Value=exp(j*2*pi*[0 -1/3 -2/3])
  Rotation1 : Constant  Value=exp(j*2*pi*[0 -1/3 -2/3])
  Square : Math  Operator=square
  Sum of Elements1 : Sum  Inputs=+
  Sum of Elements2 : Sum  Inputs=+
  Sum of Elements3 : Sum  Inputs=+
  complex_LPF : Subsystem  mask{tau=0.02}
      mask prompts: tau "Time constant"
  fund[3] : Outport
  Zero : Outport  Port=2
  Pve : Outport  Port=3
  Nve : Outport  Port=4
  wires:
  in[3]/1 -> Product1/1
  Gain2/1 -> Zero/1
  Gain3/1 -> Pve/1  "Ipve"
  osc[3]/1 -> Demux/1
  Sum of Elements3/1 -> Gain4/1
  Square/1 -> Product2/2
  Sum of Elements1/1 -> Gain2/1
  Conj/1 -> Product1/2
  Sum of Elements2/1 -> Gain3/1
  Rotation1/1 -> Product3/2
  Rotation/1 -> Square/1
  Demux/1 -> Conj/1
  Gain1/1 -> complex_LPF/1(In1)
  Product3/1 -> Sum of Elements3/1
  Product1/1 -> Gain1/1
  complex_LPF/1(Out1) -> Sum of Elements1/1, Product2/1, Product3/1
  Product2/1 -> Sum of Elements2/1, fund[3]/1
  Gain4/1 -> Nve/1

== system controls_module_lib/currentLimiting_A/excess_sink ==
  I_total[3] : Inport
  osc[3] : Inport  Port=2
  Complex to Real-Imag : ComplexToRealImag
  Ilimit : Constant  Value=RmsLimit * IRated
  Product3 : Product
  RMS Limiter : Subsystem
  Sum : Sum  Inputs=|-+
  sqrt(2) : Gain  Gain=sqrt(2)
  i_excess[3] : Outport
  wires:
  sqrt(2)/1 -> Product3/2
  Product3/1 -> Complex to Real-Imag/1
  I_total[3]/1 -> RMS Limiter/2(I[3]), Sum/2
  Sum/1 -> Product3/1  "Iexcess[3]"
  Complex to Real-Imag/1 -> i_excess[3]/1
  osc[3]/1 -> sqrt(2)/1
  Ilimit/1 -> RMS Limiter/1(limit)
  RMS Limiter/1(I_limited[3]) -> Sum/1

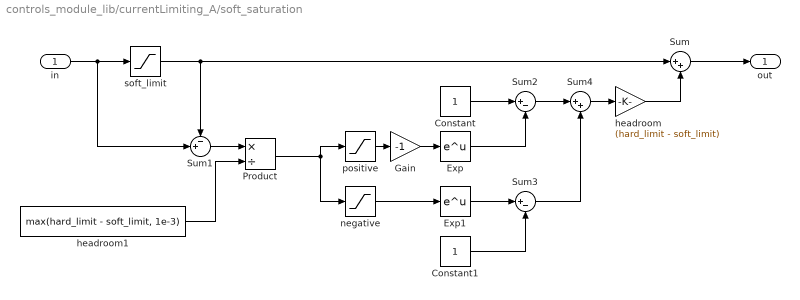
== system controls_module_lib/currentLimiting_A/soft_saturation ==
  in : Inport
  Constant : Constant
  Constant1 : Constant
  Exp : Math
  Exp1 : Math
  Gain : Gain  Gain=-1
  Product : Product  Inputs=*/
  Sum : Sum  Inputs=|++
  Sum1 : Sum  Inputs=-+|
  Sum2 : Sum  Inputs=|+-
  Sum3 : Sum  Inputs=|+-
  Sum4 : Sum  Inputs=|++
  headroom : Gain  Gain=(hard_limit - soft_limit)
  headroom1 : Constant  Value=max(hard_limit - soft_limit, 1e-3)
  negative : Saturate  UpperLimit=0  LowerLimit=-inf
  positive : Saturate  UpperLimit=inf  LowerLimit=0
  soft_limit : Saturate  UpperLimit=soft_limit  LowerLimit=-soft_limit
  out : Outport
  wires:
  Constant/1 -> Sum2/1
  Product/1 -> negative/1, positive/1
  Constant1/1 -> Sum3/2
  negative/1 -> Exp1/1
  Sum3/1 -> Sum4/2
  soft_limit/1 -> Sum/1, Sum1/1
  Sum/1 -> out/1
  Exp1/1 -> Sum3/1
  in/1 -> Sum1/2, soft_limit/1
  positive/1 -> Gain/1
  Exp/1 -> Sum2/2
  headroom/1 -> Sum/2
  Gain/1 -> Exp/1
  Sum4/1 -> headroom/1
  Sum2/1 -> Sum4/1
  Sum1/1 -> Product/1
  headroom1/1 -> Product/2

== system controls_module_lib/currentSource_A/LVRT_foldback ==
  Vpve_pu : Inport
  Complex to Magnitude-Angle : ComplexToMagnitudeAngle
  Constant1 : Constant
  Gain : Gain  Gain=3
  Saturation : Saturate  UpperLimit=Plimit  LowerLimit=0.05
  Sum1 : Sum  Inputs=|+-
  Sum2 : Sum  Inputs=|++
  Transfer Fcn : TransferFcn  Denominator=[0.02 1]
  foldback_threshold : Constant  Value=0.4
  limit_pu : Outport
  wires:
  Sum1/1 -> Transfer Fcn/1
  Gain/1 -> Sum2/1
  Transfer Fcn/1 -> Gain/1
  Complex to Magnitude-Angle/1 -> Sum1/1
  Sum2/1 -> Saturation/1
  Constant1/1 -> Sum2/2
  foldback_threshold/1 -> Sum1/2
  Vpve_pu/1 -> Complex to Magnitude-Angle/1
  Saturation/1 -> limit_pu/1

== system controls_module_lib/currentSource_A/current_modulator ==
  I_cmd : Inport
  osc : Inport  Port=2
  Complex to Real-Imag : ComplexToRealImag
  Complex to Real-Imag1 : ComplexToRealImag
  Gain : Gain  Gain=sqrt(2)
  Product1 : Product
  Product2 : Product
  Sum1 : Sum  Inputs=|+-
  i_ref : Outport
  wires:
  osc/1 -> Gain/1
  Complex to Real-Imag/1 -> Product2/2
  Product2/1 -> Sum1/1
  Sum1/1 -> i_ref/1  "i"
  Gain/1 -> Complex to Real-Imag/1
  Complex to Real-Imag/2 -> Product1/2
  Product1/1 -> Sum1/2
  I_cmd/1 -> Complex to Real-Imag1/1
  Complex to Real-Imag1/1 -> Product2/1
  Complex to Real-Imag1/2 -> Product1/1

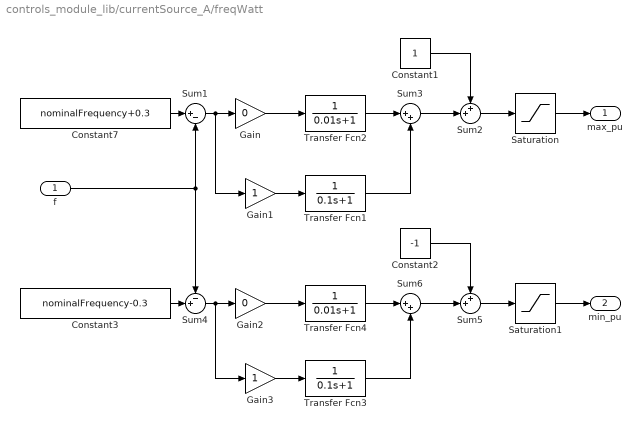
== system controls_module_lib/currentSource_A/freqWatt ==
  f : Inport
  Constant1 : Constant
  Constant2 : Constant  Value=-1
  Constant3 : Constant  Value=nominalFrequency-0.3
  Constant7 : Constant  Value=nominalFrequency+0.3
  Gain : Gain  Gain=0
  Gain1 : Gain
  Gain2 : Gain  Gain=0
  Gain3 : Gain
  Saturation : Saturate  UpperLimit=Plimit  LowerLimit=0.05
  Saturation1 : Saturate  UpperLimit=-0.05  LowerLimit=-Plimit
  Sum1 : Sum  Inputs=|+-
  Sum2 : Sum  Inputs=++|
  Sum3 : Sum  Inputs=|++
  Sum4 : Sum  Inputs=-+|
  Sum5 : Sum  Inputs=++|
  Sum6 : Sum  Inputs=|++
  Transfer Fcn1 : TransferFcn  Denominator=[0.1 1]
  Transfer Fcn2 : TransferFcn  Denominator=[0.01 1]
  Transfer Fcn3 : TransferFcn  Denominator=[0.1 1]
  Transfer Fcn4 : TransferFcn  Denominator=[0.01 1]
  max_pu : Outport
  min_pu : Outport  Port=2
  wires:
  Gain/1 -> Transfer Fcn2/1
  Constant7/1 -> Sum1/1
  Sum1/1 -> Gain1/1, Gain/1
  Constant1/1 -> Sum2/1
  Sum3/1 -> Sum2/2
  f/1 -> Sum4/1, Sum1/2
  Sum2/1 -> Saturation/1
  Transfer Fcn2/1 -> Sum3/1
  Gain1/1 -> Transfer Fcn1/1
  Transfer Fcn1/1 -> Sum3/2
  Saturation/1 -> max_pu/1
  Saturation1/1 -> min_pu/1
  Transfer Fcn3/1 -> Sum6/2
  Gain3/1 -> Transfer Fcn3/1
  Transfer Fcn4/1 -> Sum6/1
  Sum5/1 -> Saturation1/1
  Sum6/1 -> Sum5/2
  Constant2/1 -> Sum5/1
  Sum4/1 -> Gain2/1, Gain3/1
  Constant3/1 -> Sum4/2
  Gain2/1 -> Transfer Fcn4/1

== system controls_module_lib/dc voltage regulator/SOGI ==
  in : Inport
  fnom : Inport  Port=2
  2pi : Gain  Gain=2*pi
  Integrator2 : Integrator
  Integrator3 : Integrator
  Product : Product
  Product1 : Product
  Sum4 : Sum  Inputs=|+-
  Sum5 : Sum  Inputs=|+-
  alpha : Gain  Gain=0.1
  notch : Outport
  bpf : Outport  Port=2
  wires:
  Product1/1 -> Integrator3/1
  Product/1 -> Integrator2/1
  2pi/1 -> Product/2, Product1/2
  Integrator3/1 -> Sum4/2
  Sum4/1 -> Product/1
  Sum5/1 -> notch/1, alpha/1
  alpha/1 -> Sum4/1
  Integrator2/1 -> bpf/1, Sum5/2, Product1/1
  fnom/1 -> 2pi/1
  in/1 -> Sum5/1

== system controls_module_lib/machineModel_A/assymmetric filter1 ==
  note: The saturation block is configured to cause a rapid rise, but much slow drop in output.
  in : Inport
  Gain1 : Gain  Gain=2
  Integrator : Integrator
  Saturation1 : Saturate  UpperLimit=1  LowerLimit=-0.02
  Sum3 : Sum  Inputs=|+-
  out : Outport
  wires:
  Integrator/1 -> out/1, Sum3/2
  Sum3/1 -> Gain1/1
  in/1 -> Sum3/1
  Gain1/1 -> Saturation1/1
  Saturation1/1 -> Integrator/1

== system controls_module_lib/machineModel_A/excitation ==
  note: This limit is needed to avoid excessive currents during blackstart that cause windup in current limiting logic.. It results in a linear ramp of voltage during blackstart
  Vemf : Inport
  osc[3] : Inport  Port=2
  V+_conditioned_pu : Inport  Port=3
  Complex to Real-Imag : ComplexToRealImag
  Gain2 : Gain  Gain=1/sqrt(3)
  LPF : TransferFcn  Denominator=[0.1 1]
  Min : MinMax  Inputs=2
  Product1 : Product
  Saturation1 : Saturate  UpperLimit=1.1*VllRated  LowerLimit=0.9*VllRated
  Sum : Sum  Inputs=|++
  sqrt(2) : Gain  Gain=sqrt(2)
  to_SI : Gain  Gain=VllRated
  voltage_headroom : Constant  Value=0.3*VllRated
  v_emf : Outport
  wires:
  Product1/1 -> sqrt(2)/1
  Complex to Real-Imag/1 -> Product1/2
  osc[3]/1 -> Complex to Real-Imag/1
  Gain2/1 -> Product1/1  "Vref_LN"
  sqrt(2)/1 -> v_emf/1
  Vemf/1 -> Saturation1/1
  Min/1 -> LPF/1
  V+_conditioned_pu/1 -> to_SI/1
  LPF/1 -> Gain2/1
  voltage_headroom/1 -> Sum/2
  Saturation1/1 -> Min/1
  Sum/1 -> Min/2
  to_SI/1 -> Sum/1

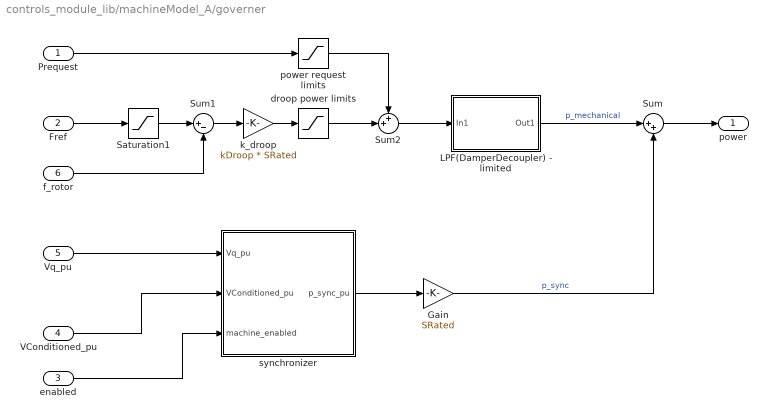
== system controls_module_lib/machineModel_A/governer ==
  Prequest : Inport
  Fref : Inport  Port=2
  enabled : Inport  Port=3
  VConditioned_pu : Inport  Port=4
  Vq_pu : Inport  Port=5
  f_rotor : Inport  Port=6
  Gain : Gain  Gain=SRated
  LPF(DamperDecoupler) - limited : Subsystem
  Saturation1 : Saturate  UpperLimit=nominalFrequency+1  LowerLimit=nominalFrequency-1
  Sum : Sum  Inputs=|++
  Sum1 : Sum  Inputs=|+-
  Sum2 : Sum  Inputs=++|
  droop power limits : Saturate  UpperLimit=SRated  LowerLimit=-SRated
  k_droop : Gain  Gain=kDroop * SRated
  power request limits : Saturate  UpperLimit=SRated  LowerLimit=-SRated
  synchronizer : Subsystem
  power : Outport
  wires:
  Sum1/1 -> k_droop/1
  synchronizer/1(p_sync_pu) -> Gain/1
  Sum/1 -> power/1
  Fref/1 -> Saturation1/1
  f_rotor/1 -> Sum1/2
  Saturation1/1 -> Sum1/1
  LPF(DamperDecoupler) - limited/1(Out1) -> Sum/1  "p_mechanical"
  VConditioned_pu/1 -> synchronizer/2(VConditioned_pu)
  enabled/1 -> synchronizer/3(machine_enabled)
  Sum2/1 -> LPF(DamperDecoupler) - limited/1(In1)
  k_droop/1 -> droop power limits/1
  Prequest/1 -> power request limits/1
  Vq_pu/1 -> synchronizer/1(Vq_pu)
  Gain/1 -> Sum/2  "p_sync"
  droop power limits/1 -> Sum2/2
  power request limits/1 -> Sum2/1

== system controls_module_lib/machineModel_A/impedance_emulation ==
  v_emf : Inport
  v_terminal : Inport  Port=2
  enable : Inport  Port=3
  Constant : Constant  Value=0
  Integrator : Integrator
  Sum : Sum  Inputs=|+-
  Sum of Elements1 : Sum  Inputs=+
  Sum1 : Sum  Inputs=|+-
  Sum4 : Sum  Inputs=|+-
  Switch : Switch  Criteria=u2 > Threshold  SaturateOnIntegerOverflow=off  InputSameDT=off
  overLs : Gain  Gain=2*pi*60/(Xs * (VllRated^2/SRated))
  rN : Gain  Gain=0.2*(VllRated^2/SRated)
  rs : Gain  Gain=rs*(VllRated^2/SRated)
  i_ref : Outport
  wires:
  Integrator/1 -> i_ref/1, rs/1, Sum of Elements1/1  "i_ref"
  rs/1 -> Sum1/2
  rN/1 -> Sum4/2
  Sum1/1 -> overLs/1
  Sum4/1 -> Sum1/1
  Sum of Elements1/1 -> rN/1
  overLs/1 -> Integrator/1
  v_emf/1 -> Sum/1
  v_terminal/1 -> Sum/2
  Switch/1 -> Sum4/1
  Sum/1 -> Switch/1
  Constant/1 -> Switch/3
  enable/1 -> Switch/2

== system controls_module_lib/machineModel_A/rotor model ==
  p_mechanical : Inport
  p_electrical : Inport  Port=2
  Constant : Constant  Value=nominalFrequency
  HPF (wDamperDecoupler) : TransferFcn  Numerator=[0.3 0]  Denominator=[0.3 1]
  Integrator1 : Integrator  LimitOutput=on  UpperSaturationLimit=5  LowerSaturationLimit=-5
  Sum : Sum  Inputs=++|
  Sum2 : Sum  Inputs=|+-
  Sum3 : Sum  Inputs=|+-
  k_damp : Gain  Gain=kDamper*SRated
  k_inertia : Gain  Gain=(nominalFrequency/2)/(inertialConstant*SRated)
  oscillator_3ph : Subsystem
  osc[3] : Outport
  f : Outport  Port=2
  wires:
  Sum2/1 -> k_inertia/1
  k_inertia/1 -> Integrator1/1
  oscillator_3ph/1(osc[3]) -> osc[3]/1
  HPF (wDamperDecoupler)/1 -> k_damp/1
  p_electrical/1 -> Sum3/2
  Sum3/1 -> Sum2/1
  p_mechanical/1 -> Sum3/1
  Integrator1/1 -> Sum/2, HPF (wDamperDecoupler)/1
  k_damp/1 -> Sum2/2
  Sum/1 -> f/1, oscillator_3ph/1(f)
  Constant/1 -> Sum/1

== system controls_module_lib/machineModel_A/voltage_analyzer ==
  osc[3] : Inport
  v_pu : Inport  Port=2
  Complex to Real-Imag : ComplexToRealImag
  Conj : Math  Operator=conj
  Product1 : Product
  Product2 : Product
  Sum of Elements1 : Sum  Inputs=+
  Sum of Elements2 : Sum  Inputs=+
  Transfer Fcn : TransferFcn  Denominator=[0.02 1]
  Transfer Fcn1 : TransferFcn  Denominator=[0.02 1]
  over_sqrt(3) : Gain  Gain=1/sqrt(3)
  over_sqrt(3)1 : Gain  Gain=1/sqrt(3)
  sqrt(2) : Gain  Gain=sqrt(2)
  Vq_pu : Outport
  Vd_pu : Outport  Port=2
  wires:
  Product2/1 -> Sum of Elements2/1
  Conj/1 -> sqrt(2)/1
  sqrt(2)/1 -> Complex to Real-Imag/1
  Sum of Elements1/1 -> over_sqrt(3)/1
  Product1/1 -> Sum of Elements1/1
  v_pu/1 -> Product1/2, Product2/2
  Sum of Elements2/1 -> over_sqrt(3)1/1
  Complex to Real-Imag/2 -> Product1/1
  Complex to Real-Imag/1 -> Product2/1
  over_sqrt(3)/1 -> Transfer Fcn/1
  over_sqrt(3)1/1 -> Transfer Fcn1/1
  Transfer Fcn1/1 -> Vd_pu/1  "Vd_pu"
  osc[3]/1 -> Conj/1
  Transfer Fcn/1 -> Vq_pu/1  "Vq_pu"

== system controls_module_lib/acMonitor_A/Analyzer_V/complex_LPF ==
  note: This was needed because Simulink complains when using transfer functions directly on arrays or complex numbers.
  In1 : Inport
  Complex to Real-Imag : ComplexToRealImag
  Gain2 : Gain  Gain=1/tau
  Gain3 : Gain  Gain=1/tau
  Integrator : Integrator
  Integrator1 : Integrator
  Real-Imag to Complex : RealImagToComplex
  Sum : Sum  Inputs=|+-
  Sum1 : Sum  Inputs=|+-
  Out1 : Outport
  wires:
  Real-Imag to Complex/1 -> Out1/1
  In1/1 -> Complex to Real-Imag/1
  Complex to Real-Imag/1 -> Sum/1
  Integrator/1 -> Real-Imag to Complex/1, Sum/2
  Sum1/1 -> Gain3/1
  Complex to Real-Imag/2 -> Sum1/1
  Gain2/1 -> Integrator/1
  Sum/1 -> Gain2/1
  Integrator1/1 -> Sum1/2, Real-Imag to Complex/2
  Gain3/1 -> Integrator1/1

== system controls_module_lib/acMonitor_A/PLL_3ph/oscillator_3ph ==
  f : Inport
  Cos : Trigonometry  Operator=cos
  Gain : Gain  Gain=2*pi
  Integrator : Integrator
  Real-Imag to Complex : RealImagToComplex
  Sin : Trigonometry
  Sum1 : Sum  Inputs=|++
  phase_shift : Constant  Value=[0 -1/3 -2/3]
  osc[3] : Outport
  wires:
  Sum1/1 -> Gain/1
  phase_shift/1 -> Sum1/2
  Sin/1 -> Real-Imag to Complex/2
  Integrator/1 -> Sum1/1
  Gain/1 -> Sin/1, Cos/1
  Cos/1 -> Real-Imag to Complex/1
  Real-Imag to Complex/1 -> osc[3]/1
  f/1 -> Integrator/1

== system controls_module_lib/currentLimiting_A/Analyzer_I/complex_LPF ==
  note: This was needed because Simulink complains when using transfer functions directly on arrays or complex numbers.
  In1 : Inport
  Complex to Real-Imag : ComplexToRealImag
  Gain2 : Gain  Gain=1/tau
  Gain3 : Gain  Gain=1/tau
  Integrator : Integrator
  Integrator1 : Integrator
  Real-Imag to Complex : RealImagToComplex
  Sum : Sum  Inputs=|+-
  Sum1 : Sum  Inputs=|+-
  Out1 : Outport
  wires:
  Real-Imag to Complex/1 -> Out1/1
  In1/1 -> Complex to Real-Imag/1
  Complex to Real-Imag/1 -> Sum/1
  Integrator/1 -> Real-Imag to Complex/1, Sum/2
  Sum1/1 -> Gain3/1
  Complex to Real-Imag/2 -> Sum1/1
  Gain2/1 -> Integrator/1
  Sum/1 -> Gain2/1
  Integrator1/1 -> Sum1/2, Real-Imag to Complex/2
  Gain3/1 -> Integrator1/1

== system controls_module_lib/currentLimiting_A/excess_sink/RMS Limiter ==
  limit : Inport
  I[3] : Inport  Port=2
  Abs1 : Abs  SaturateOnIntegerOverflow=off
  Max : MinMax  Function=max
  Min : MinMax  Function=max  Inputs=2
  Product1 : Product  Inputs=*/
  Product2 : Product
  I_limited[3] : Outport
  wires:
  Product2/1 -> I_limited[3]/1
  Min/1 -> Product1/2
  Max/1 -> Min/2  "highest phase current"
  Product1/1 -> Product2/1  "scale_factor"
  Abs1/1 -> Max/1
  I[3]/1 -> Product2/2, Abs1/1
  limit/1 -> Product1/1, Min/1

== system controls_module_lib/machineModel_A/governer/LPF(DamperDecoupler) - limited ==
  In1 : Inport
  Integrator : Integrator  LimitOutput=on  UpperSaturationLimit=1.2*SRated  LowerSaturationLimit=-1.2*SRated
  Sum3 : Sum  Inputs=|+-
  wDamperDecoupler : Gain  Gain=3.33
  Out1 : Outport
  wires:
  In1/1 -> Sum3/1
  wDamperDecoupler/1 -> Integrator/1
  Sum3/1 -> wDamperDecoupler/1
  Integrator/1 -> Sum3/2, Out1/1
